simulink model "vehicle_ice"  (R2017a)
settings: Solver=FixedStepDiscrete  StartTime=0.0  StopTime=inf  FixedStep=abs(Ts)  RelTol=1e-3
InitFcn:
  | if ~exist('Ts')
  |     Ts = 1;
  | end
undefined symbols (not defined in the file or in its folder): elvio_cycle_wltp_3b
libraries: elvio x11
settings Model: Creator=tstef  LastModifiedBy=elts2

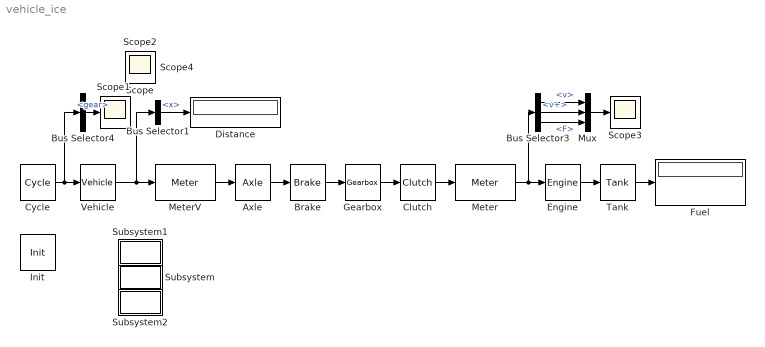
== system vehicle_ice ==
  Axle : elvio/Drive/Axle  radius=0.3  ratio=4  factor=0.1  FromTag1=Axle1  GotoTag1=MeterV1
  Brake : elvio/Drive/Brake  Tbrake=5000  FromTag1=Brake1  GotoTag1=Axle1
  Bus Selector1 : BusSelector  OutputSignals=info.x
  Bus Selector3 : BusSelector  OutputSignals=v,v+,F
  Bus Selector4 : BusSelector  OutputSignals=gear
  Clutch : elvio/Drive/Clutch  speed=70  FromTag1=Clutch1  GotoTag1=Gearbox1
  Cycle : elvio/Drive/Cycle  data=elvio_cycle_wltp_3b()  acc=-3
  Distance : Display
  Engine : elvio/Drive/Engine  Tmax=110  Tmin=0  Tfrict=16  Ploss=800  lossf=0.8  lossnorm=125e3  lossR=0.25  FromTag1=Engine1  GotoTag1=Meter1
  Fuel : Display
  Gearbox : elvio/Drive/Gearbox  gears=[4 2.5 1.8 1.2 0.9 0.9]  factor=0.1  FromTag1=Gearbox1  GotoTag1=Brake1
  Init : elvio/Drive/Init  Ts0=1
  Meter : elvio/Drive/Meter  d=100  FromTag1=Meter1  GotoTag1=Clutch1
  MeterV : elvio/Drive/Meter  d=100  FromTag1=MeterV1  GotoTag1=Vehicle1
  Mux : Mux  Inputs=3
  Scope{,1..4} (5 alike) : Scope
      Scope4 mask Display: disp('1.484e+07')
  Subsystem : Subsystem
      settings: OpenFcn=elvio_plot_scatter(logsout);
      mask Display: disp('Scatter')
  Subsystem1 : Subsystem
      settings: OpenFcn=elvio_plot_energy(logsout);
      mask Display: disp('Energy')
  Subsystem2 : Subsystem
      settings: OpenFcn=elvio_plot_sources(logsout);
      mask Display: disp('Sources')
  Tank : elvio/Drive/Tank  GotoTag1=Engine1
  Vehicle : elvio/Drive/Vehicle  m=1200  Froll=150  Aeff=0.3  n=[1 5]  FromTag1=Vehicle1
  wires:
  Vehicle/1 -> MeterV/1, Bus Selector1/1
  Engine/1 -> Tank/1
  Tank/1 -> Fuel/1
  Gearbox/1 -> Clutch/1
  Bus Selector1/1 -> Distance/1  "<x>"
  MeterV/1 -> Axle/1
  Bus Selector3/3 -> Mux/3  "<F>"
  Bus Selector3/2 -> Mux/2  "<v+>"
  Mux/1 -> Scope3/1
  Meter/1 -> Engine/1, Bus Selector3/1
  Bus Selector3/1 -> Mux/1  "<v>"
  Cycle/1 -> Vehicle/1, Bus Selector4/1
  Bus Selector4/1 -> Scope1/1  "<gear>"
  Axle/1 -> Brake/1
  Brake/1 -> Gearbox/1
  Clutch/1 -> Meter/1

== system vehicle_ice/Subsystem ==

== system vehicle_ice/Subsystem1 ==

== system vehicle_ice/Subsystem2 ==
